simulink model "s3b"  (Simulink 2.00)
settings: Solver=ode15s  StartTime=0.0  StopTime=140  MaxStep=0.1  RelTol=1e-6  AbsTol=1e-6
values from neighbouring files (symbols this model uses):
  Iarated = 16    [M1.M]    (also in M2.M = 33.9090909091; M3A.M; M3B.M; M4.M = 3.5)
  J = 0.8    [M1.M]    (also in M2.M = 2.5; M3A.M = 0.5; M3B.M = 0.5; M4.M = 0.015)
  Laq = 0.018    [M1.M]    (also in M2.M = 0.012; M3A.M; M3B.M; M4.M = 0.01)
  Ra = 0.24    [M1.M]    (also in M2.M = 0.3; M3A.M = 0.14; M3B.M = 0.14; M4.M = 0.6)
  Trated = Prated/wmrated    (= 8.14145743176)    [M1.M]    (also in M2.M = 47.8105721664; M3A.M; M3B.M; M4.M = 1.10840049653)
  wlower = -wmrated/3    (= -61.0865238198)    [M3B.M]
  wraise = wmrated    (= 183.259571459)    [M3B.M]
settings Model: SaveTime=off  SaveOutput=off  ConsistencyChecking=off

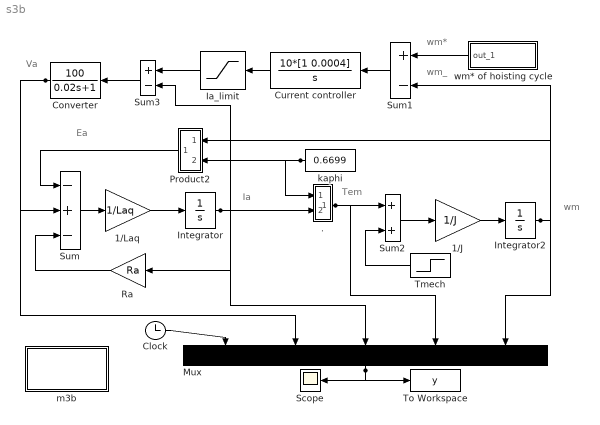
== system s3b ==
  note: Ia
  note: Tem
  note: Ea
  note: wm*
  note: wm_
  note: Va
  note: wm
  . : Subsystem
      mask Type: Dot Product
      mask Description:
      | Inner (dot) product.
      | y=sum(u1.*u2)
      mask Help: Computes the inner (dot) product of the inputs: sum(u1.*u2).  The inputs are vectors of the same length. Output is a scalar.
      mask Display: disp('.\n')
  1/J : Gain  Gain=1/J
  1/Laq : Gain  Gain=1/Laq
  Clock : Clock
      settings: DeleteFcn=simclock BlockIsBeingDestroyed  PostSaveFcn=simclock Save
  Converter : TransferFcn  Orientation=left  Numerator=[100]  Denominator=[0.02 1]
  Current controller : TransferFcn  Orientation=left  Numerator=10*[1 0.0004]  Denominator=[1 0 ]
  Ia_limit : Saturate  Orientation=left  UpperLimit=Iarated*1.2  LowerLimit=-Iarated*1.2
  Integrator : Integrator  ExternalReset=none  InitialConditionSource=internal  InitialCondition=0  LimitOutput=off  UpperSaturationLimit=inf  LowerSaturationLimit=-inf  ShowSaturationPort=off  ShowStatePort=off  AbsoluteTolerance=auto
  Integrator2 : Integrator  ExternalReset=none  InitialConditionSource=internal  InitialCondition=0  LimitOutput=off  UpperSaturationLimit=inf  LowerSaturationLimit=-inf  ShowSaturationPort=off  ShowStatePort=off  AbsoluteTolerance=auto
  m3b : Subsystem
      settings: OpenFcn=m3b
      mask Type: Masked block of m3b.m
      mask Help: Uses m3b.m to initialize and plot
      mask Display: disp('Initialize\nand plot')
  Mux : Mux  Orientation=down  Inputs=5
  Product2 : Subsystem  Orientation=left
      mask Type: Dot Product
      mask Description:
      | Inner (dot) product.
      | y=sum(u1.*u2)
      mask Help: Computes the inner (dot) product of the inputs: sum(u1.*u2).  The inputs are vectors of the same length. Output is a scalar.
      mask Display: disp('.\n')
  Ra : Gain  Orientation=left  Gain=Ra
  Scope : Scope
      settings: TickLabels=on  TimeRange=150  YMin=-200  YMax=200  SaveToWorkspace=off  SaveName=ScopeData  LimitMaxRows=off
  Sum : Sum  Inputs=-+-
  Sum1 : Sum  Orientation=left  Inputs=+-
  Sum2 : Sum  Inputs=++
  Sum3 : Sum  Orientation=left  Inputs=+-
  Tmech : Step  Orientation=left  Time=1  Before=0  After=-Trated
  To Workspace : ToWorkspace  VariableName=y  SampleTime=0
      settings: Buffer=30000
  kaphi : Constant  Orientation=left  Value=0.6699
  wm* of hoisting cycle : Subsystem  Orientation=left  mask(Repeating table){rep_seq_t=[0 30 40  50  65 75 85 95 100], rep_seq_y=[0 wraise wraise 0 0 wlower wlower 0 0]}
      mask prompts: rep_seq_t "Time values:"; rep_seq_y "Output values:"
      mask help: Repeating table.
      mask init:
      | period = max(rep_seq_t);
      mask Help: Repeats cycle given in table. Time values should be monotonically increasing.
      mask Display: plot([rep_seq_t,rep_seq_t+period,rep_seq_t+2*period,rep_seq_t(1)+3*period],[rep_seq_y,rep_seq_y,rep_seq_y,rep_seq_y(1)])
  wires:
  wm* of hoisting cycle/1(out_1) -> Sum1/1
  ./1(out_1) -> Mux/4, Sum2/1
  Converter/1 -> Mux/2, Sum/2
  Sum3/1 -> Converter/1
  Ia_limit/1 -> Sum3/1
  Sum1/1 -> Current controller/1
  Current controller/1 -> Ia_limit/1
  Tmech/1 -> Sum2/2
  Ra/1 -> Sum/3
  Integrator2/1 -> Mux/5, Sum1/2, Product2/1(in_1)
  kaphi/1 -> ./1(in_1), Product2/2(in_2)
  Clock/1 -> Mux/1
  Mux/1 -> Scope/1, To Workspace/1
  Integrator/1 -> Mux/3, Sum3/2, Ra/1, ./2(in_2)
  1/Laq/1 -> Integrator/1
  Product2/1(out_1) -> Sum/1
  1/J/1 -> Integrator2/1
  Sum2/1 -> 1/J/1
  Sum/1 -> 1/Laq/1

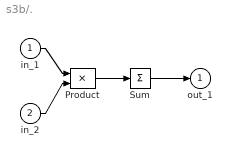
== system s3b/. ==
  in_1 : Inport  Port=1  PortWidth=-1  SampleTime=-1
  in_2 : Inport  Port=2  PortWidth=-1  SampleTime=-1
  Product : Product  Inputs=2
  Sum : Sum  Inputs=+
  out_1 : Outport  Port=1  InitialOutput=0
  wires:
  Sum/1 -> out_1/1
  Product/1 -> Sum/1
  in_1/1 -> Product/1
  in_2/1 -> Product/2

== system s3b/m3b ==
  note: Masked block of m3b.m to initialize
      | s3b.m and plot results

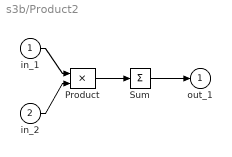
== system s3b/Product2 ==
  in_1 : Inport  Port=1  PortWidth=-1  SampleTime=-1
  in_2 : Inport  Port=2  PortWidth=-1  SampleTime=-1
  Product : Product  Inputs=2
  Sum : Sum  Inputs=+
  out_1 : Outport  Port=1  InitialOutput=0
  wires:
  Sum/1 -> out_1/1
  Product/1 -> Sum/1
  in_1/1 -> Product/1
  in_2/1 -> Product/2

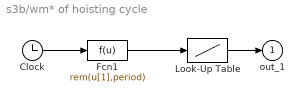
== system s3b/wm* of hoisting cycle ==
  Clock : Clock
      settings: DeleteFcn=simclock BlockIsBeingDestroyed  PostSaveFcn=simclock Save
  Fcn1 : Fcn  Expr=rem(u[1],period)
  Look-Up Table : Lookup  InputValues=rep_seq_t  OutputValues=rep_seq_y
  out_1 : Outport  Port=1  InitialOutput=0
  wires:
  Look-Up Table/1 -> out_1/1
  Clock/1 -> Fcn1/1
  Fcn1/1 -> Look-Up Table/1
